simulink model "TestBulk"  (R2018a)
settings: Solver=VariableStepAuto  StartTime=0.0  StopTime=10  FixedStep=0.2  RelTol=1e-3  EnableMultiTasking=on
settings Model: SimulationMode=accelerator  EnablePacing=on  Creator=Hungs  LastModifiedBy=Hungs

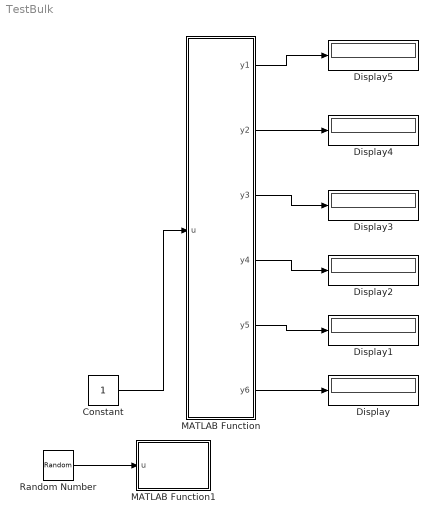
== system TestBulk ==
  Constant : Constant
  Display{,1..5} (6 alike) : Display
      settings: Decimation=2
  MATLAB Function : MATLAB Function  TreatAsAtomicUnit=on
  MATLAB Function1 : MATLAB Function  TreatAsAtomicUnit=on
  Random Number : RandomNumber  Mean=5  Variance=5
  wires:
  MATLAB Function/1(y1) -> Display5/1
  Random Number/1 -> MATLAB Function1/1(u)
  Constant/1 -> MATLAB Function/1(u)
  MATLAB Function/2(y2) -> Display4/1
  MATLAB Function/3(y3) -> Display3/1
  MATLAB Function/4(y4) -> Display2/1
  MATLAB Function/5(y5) -> Display1/1
  MATLAB Function/6(y6) -> Display/1

== matlab function TestBulk/MATLAB Function ==
  data: u input; y1 output; y2 output; y3 output; y4 output; y5 output; y6 output
function [y1,y2,y3,y4,y5,y6] = fcn(u)
coder.extrinsic('AdsReadBulk');
y1 = int16(0);
y2 = int32(0);
y3 = int32(0);
y4 = int8(0);
y5 = single(0);
y6 = double(0);
if u==1
    [y1, y2, y3, y4, y5, y6] = AdsReadBulk();
end
end

== matlab function TestBulk/MATLAB Function1 ==
  data: u input
function fcn(u)
coder.extrinsic('AdsWriteBulk');
    AdsWriteBulk( u);
end
